simulink library "SimscapeCustomComponents_lib"  (R2025b)
settings: Solver=VariableStepAuto  StartTime=0.0  StopTime=10.0  RelTol=1e-3
undefined symbols (not defined in the file or in its folder): base, baseVdc, capacity, DiscIntNeverNeededParam, ee_sli_rtmsupport, filterInductance, freqeuncy, frequency, gcbh, gflInverter, gfmInverter, iMaxPU, Inertia, initialSOC, plantRating, solar, Ts, ups, Vac, windSystem, windTurbine
libraries: fl_lib x397, nesl_utility x171, eeGeneralControl x85, ee_lib x82, simulink x72, datacenter_lib x68, eeTransforms x38, slpidlib x24, buildingEnergy_lib x20, SimscapeFluids_lib x17, eeSinusoidalMeasurementV2 x8, eePwmGenerator x8
(part 17 of 24)

== system SimscapeCustomComponents_lib/Microgrid and Renewables/Control/Renewables/Power Reference Controller/PLL & Measurements/Subsystem ==
  Vabc : Inport
  Iabc : Inport  Port=2
  Demux : Demux  Outputs=3
  Demux1 : Demux  Outputs=3
  Park Transform : eeTransforms/Park Transform  AxisAlignment=Q-axis  PowerInvariant=off
  Park Transform1 : eeTransforms/Park Transform  AxisAlignment=Q-axis  PowerInvariant=off
  Scope : Scope  NumInputPorts=2
      settings: ActiveDisplayYMinimum=0.97158  ActiveDisplayYMaximum=1.00612  DataLoggingVariableName=ScopeData5
  "Sinusoidal Measurement (PLL, Three-Phase)" : eeSinusoidalMeasurementV2/Sinusoidal Measurement (PLL, Three-Phase)  InputFilter=on  InputNormalization=off  Kp_LF=kpPLL  Ki_LF=kiPLL  F0=frequency  Theta0=0  Ts=-1
  Terminator : Terminator
  Terminator1 : Terminator
  mag : Outport
  freq : Outport  Port=2
  angle : Outport  Port=3
  Vd : Outport  Port=4
  Vq : Outport  Port=5
  Id1 : Outport  Port=6
  Iq1 : Outport  Port=7
  wires:
  Demux/3 -> Terminator/1
  Vabc/1 -> Park Transform/1, "Sinusoidal Measurement (PLL, Three-Phase)"/1
  Park Transform/1 -> Demux/1
  Demux/1 -> Scope/1, Vd/1
  Demux/2 -> Scope/2, Vq/1
  "Sinusoidal Measurement (PLL, Three-Phase)"/2 -> angle/1, Park Transform1/2, Park Transform/2
  "Sinusoidal Measurement (PLL, Three-Phase)"/1 -> freq/1
  "Sinusoidal Measurement (PLL, Three-Phase)"/3 -> mag/1
  Park Transform1/1 -> Demux1/1
  Demux1/1 -> Id1/1
  Demux1/2 -> Iq1/1
  Demux1/3 -> Terminator1/1
  Iabc/1 -> Park Transform1/1

== system SimscapeCustomComponents_lib/Microgrid and Renewables/Control/Renewables/Power Reference Controller/Power Reference Controller/Current_controller ==
  id-ref : Inport
  ipvd : Inport  Port=2
  iqref : Inport  Port=3
  iq : Inport  Port=4
  Vd : Inport  Port=5
  Vq : Inport  Port=6
  Constant4 : Constant  Value=0
  Gain1 : Gain  Gain=2*1*pi*60*L/zbase
  Gain2 : Gain  Gain=2*1*pi*60*L/zbase
  Mux1 : Mux  Inputs=3
  PID Controller : slpidlib/PID Controller  Controller=PID  Form=Parallel  TimeDomain=Discrete-time  UseExternalTs=off  SampleTime=-1  IntegratorMethod=Forward Euler  FilterMethod=Forward Euler  ControllerParametersSource=internal  P=Kpic  I=Kiic  UseKiTs=off  D=Kd  UseExternalDerivativeSource=off  N=100  UseFilter=on  TunerSelectOption=Transfer Function Based (PID Tuner App)  InitialConditionSource=internal  InitialConditionForIntegrator=0  InitialConditionForFilter=0  DifferentiatorICPrevScaledInput=0  ExternalReset=none  TrackingMode=off  Kt=1  LimitOutput=on  SatLimitsSource=internal  UpperSaturationLimit=3  LowerSaturationLimit=-3  LinearizeAsGain=on  AntiWindupMode=clamping  Kb=1  LimitIntegrator=on  UpperIntegratorSaturationLimit=3  LowerIntegratorSaturationLimit=-3  POutMin=[]  POutMax=[]  IOutMin=[]  IOutMax=[]  DOutMin=[]  DOutMax=[]  NOutMin=[]  NOutMax=[]  SumOutMin=[]  SumOutMax=[]  SaturationOutMin=[]  SaturationOutMax=[]  PParamMin=[]  PParamMax=[]  IParamMin=[]  IParamMax=[]  DParamMin=[]  DParamMax=[]  NParamMin=[]  NParamMax=[]  KbParamMin=[]  KbParamMax=[]  KtParamMin=[]  KtParamMax=[]  KbOutMin=[]  KbOutMax=[]  KtOutMin=[]  KtOutMax=[]  IntegratorOutMin=[]  IntegratorOutMax=[]  FilterOutMin=[]  FilterOutMax=[]  SumI1OutMin=[]  SumI1OutMax=[]  SumI2OutMin=[]  SumI2OutMax=[]  SumI3OutMin=[]  SumI3OutMax=[]  SumI4OutMin=[]  SumI4OutMax=[]  SumDOutMin=[]  SumDOutMax=[]  DifferentiatorOutMin=[]  DifferentiatorOutMax=[]  FilterDiffOutCoefMin=[]  FilterDiffOutCoefMax=[]  ReciprocalOutMin=[]  ReciprocalOutMax=[]  SumDenOutMin=[]  SumDenOutMax=[]  SumNumOutMin=[]  SumNumOutMax=[]  DivideOutMin=[]  DivideOutMax=[]  UdiffTsProdOutMin=[]  UdiffTsProdOutMax=[]  NTsProdOutMin=[]  NTsProdOutMax=[]  UintegralTsProdOutMin=[]  UintegralTsProdOutMax=[]  UngainTsProdOutMin=[]  UngainTsProdOutMax=[]  ClampingZeroOutDataTypeStr=Inherit: Inherit via back propagation  ClampingZeroOutMin=[]  ClampingZeroOutMax=[]  FilterDenConstantOutDataTypeStr=Inherit: Inherit via back propagation  FilterDenConstantOutMin=[]  FilterDenConstantOutMax=[]  PCopyOutDataTypeStr=Inherit: Inherit via back propagation  PCopyOutMin=[]  PCopyOutMax=[]  NCopyOutDataTypeStr=Inherit: Inherit via back propagation  NCopyOutMin=[]  NCopyOutMax=[]  IntegratorContinuousStateAttributes=''  IntegratorStateMustResolveToSignalObject=off  IntegratorRTWStateStorageClass=Auto  FilterContinuousStateAttributes=''  FilterStateMustResolveToSignalObject=off  FilterRTWStateStorageClass=Auto  ParallelPVariant=InternalParameters  IdealPVariant=Disabled  IVariant=InternalParameters  DVariant=InternalParameters  IntegratorVariant=Discrete  SatVariant=Enabled  AWVariant=DiscClampingParallel  PCopyVariant=Disabled  TRVariant=Disabled  FdbkBlocksVariant=Forward  IdealPFdbkVariant=Disabled  SatFdbkVariant=Disabled  DerivativeFilterVariant=ForwardEulerFilter  NVariant=InternalParameters  NCopyVariant=Disabled  FilterICVariant=InternalICsFilter  IntegratorICVariant=InternalICs  ExternalResetVariant=Disabled  TRSumVariant=Passthrough  SumFdbkVariant=Disabled  SumVariant=Sum_PID  TsampFilterVariant=InternalTs  TsampNgainVariant=Passthrough  TsampIntegralVariant=Disabled_SignalSpec  ExternalSaturationOutDataTypeStr=Inherit: Same as second input  DerivativeSourceVariant=ErrorSignal  PreIntVariant=InternalPreInt
  PID Controller1 : slpidlib/PID Controller  Controller=PID  Form=Parallel  TimeDomain=Discrete-time  UseExternalTs=off  SampleTime=-1  IntegratorMethod=Forward Euler  FilterMethod=Forward Euler  ControllerParametersSource=internal  P=Kpic  I=Kiic  UseKiTs=off  D=Kd  UseExternalDerivativeSource=off  N=100  UseFilter=on  TunerSelectOption=Transfer Function Based (PID Tuner App)  InitialConditionSource=internal  InitialConditionForIntegrator=0  InitialConditionForFilter=0  DifferentiatorICPrevScaledInput=0  ExternalReset=none  TrackingMode=off  Kt=1  LimitOutput=on  SatLimitsSource=internal  UpperSaturationLimit=3  LowerSaturationLimit=-3  LinearizeAsGain=on  AntiWindupMode=clamping  Kb=1  LimitIntegrator=on  UpperIntegratorSaturationLimit=3  LowerIntegratorSaturationLimit=-3  POutMin=[]  POutMax=[]  IOutMin=[]  IOutMax=[]  DOutMin=[]  DOutMax=[]  NOutMin=[]  NOutMax=[]  SumOutMin=[]  SumOutMax=[]  SaturationOutMin=[]  SaturationOutMax=[]  PParamMin=[]  PParamMax=[]  IParamMin=[]  IParamMax=[]  DParamMin=[]  DParamMax=[]  NParamMin=[]  NParamMax=[]  KbParamMin=[]  KbParamMax=[]  KtParamMin=[]  KtParamMax=[]  KbOutMin=[]  KbOutMax=[]  KtOutMin=[]  KtOutMax=[]  IntegratorOutMin=[]  IntegratorOutMax=[]  FilterOutMin=[]  FilterOutMax=[]  SumI1OutMin=[]  SumI1OutMax=[]  SumI2OutMin=[]  SumI2OutMax=[]  SumI3OutMin=[]  SumI3OutMax=[]  SumI4OutMin=[]  SumI4OutMax=[]  SumDOutMin=[]  SumDOutMax=[]  DifferentiatorOutMin=[]  DifferentiatorOutMax=[]  FilterDiffOutCoefMin=[]  FilterDiffOutCoefMax=[]  ReciprocalOutMin=[]  ReciprocalOutMax=[]  SumDenOutMin=[]  SumDenOutMax=[]  SumNumOutMin=[]  SumNumOutMax=[]  DivideOutMin=[]  DivideOutMax=[]  UdiffTsProdOutMin=[]  UdiffTsProdOutMax=[]  NTsProdOutMin=[]  NTsProdOutMax=[]  UintegralTsProdOutMin=[]  UintegralTsProdOutMax=[]  UngainTsProdOutMin=[]  UngainTsProdOutMax=[]  ClampingZeroOutDataTypeStr=Inherit: Inherit via back propagation  ClampingZeroOutMin=[]  ClampingZeroOutMax=[]  FilterDenConstantOutDataTypeStr=Inherit: Inherit via back propagation  FilterDenConstantOutMin=[]  FilterDenConstantOutMax=[]  PCopyOutDataTypeStr=Inherit: Inherit via back propagation  PCopyOutMin=[]  PCopyOutMax=[]  NCopyOutDataTypeStr=Inherit: Inherit via back propagation  NCopyOutMin=[]  NCopyOutMax=[]  IntegratorContinuousStateAttributes=''  IntegratorStateMustResolveToSignalObject=off  IntegratorRTWStateStorageClass=Auto  FilterContinuousStateAttributes=''  FilterStateMustResolveToSignalObject=off  FilterRTWStateStorageClass=Auto  ParallelPVariant=InternalParameters  IdealPVariant=Disabled  IVariant=InternalParameters  DVariant=InternalParameters  IntegratorVariant=Discrete  SatVariant=Enabled  AWVariant=DiscClampingParallel  PCopyVariant=Disabled  TRVariant=Disabled  FdbkBlocksVariant=Forward  IdealPFdbkVariant=Disabled  SatFdbkVariant=Disabled  DerivativeFilterVariant=ForwardEulerFilter  NVariant=InternalParameters  NCopyVariant=Disabled  FilterICVariant=InternalICsFilter  IntegratorICVariant=InternalICs  ExternalResetVariant=Disabled  TRSumVariant=Passthrough  SumFdbkVariant=Disabled  SumVariant=Sum_PID  TsampFilterVariant=InternalTs  TsampNgainVariant=Passthrough  TsampIntegralVariant=Disabled_SignalSpec  ExternalSaturationOutDataTypeStr=Inherit: Same as second input  DerivativeSourceVariant=ErrorSignal  PreIntVariant=InternalPreInt
  Saturation : Saturate  UpperLimit=1.2  LowerLimit=-1.2
  Saturation1 : Saturate  UpperLimit=1.2  LowerLimit=-1.2
  Scope : Scope  NumInputPorts=2
      settings: ActiveDisplayYMinimum=0.49995  ActiveDisplayYMaximum=0.50039
  Scope1 : Scope  NumInputPorts=2
      settings: ActiveDisplayYMinimum=-1  ActiveDisplayYMaximum=1  DataLoggingVariableName=ScopeData2
  Scope2 : Scope  NumInputPorts=3
      settings: ActiveDisplayYMinimum=0.92426  ActiveDisplayYMaximum=1.0261  DataLoggingVariableName=ScopeData2
  Sum1 : Sum  Inputs=|+-
  Sum3 : Sum  Inputs=|++-
  Sum4 : Sum  Inputs=|+++
  Sum5 : Sum  Inputs=|+-
  mdq0 : Outport
  wires:
  PID Controller/1 -> Scope2/2, Sum3/2
  Sum3/1 -> Saturation/1, [Ed]
  Gain2/1 -> Scope2/3, Sum3/3
  ipvd/1 -> Scope/2, Gain1/1, Sum1/2
  id-ref/1 -> Scope/1, Sum1/1
  Gain1/1 -> Sum4/3
  Vq/1 -> Sum4/2
  iq/1 -> Scope1/2, Gain2/1, Sum5/2
  Sum1/1 -> PID Controller/1
  Constant4/1 -> Mux1/3
  Sum5/1 -> PID Controller1/1
  PID Controller1/1 -> Sum4/1
  Sum4/1 -> Saturation1/1, [Eq]
  Mux1/1 -> mdq0/1
  iqref/1 -> Scope1/1, Sum5/1
  Saturation/1 -> Mux1/1
  Saturation1/1 -> Mux1/2
  Vd/1 -> Scope2/1, Sum3/1

== system SimscapeCustomComponents_lib/Microgrid and Renewables/Control/Renewables/Power Reference Controller/Power Reference Controller/Reference Current ==
  note: Current Limiters
  note: Avoid division by zero during start
  V-mag : Inport
  LVRT_iq : Inport  Port=2
  PRef : Inport  Port=3
  QRef : Inport  Port=4
  Constant1 : Constant
  Constant3 : Constant  Value=Imax
  Current limits : Subsystem
  Refernce id generation : Subsystem
  Refernce iq generation : Subsystem
  Switch : Switch  Criteria=u2 ~= 0  SaturateOnIntegerOverflow=off  InputSameDT=off
  Unit Delay1 : UnitDelay  SampleTime=Ts
  Unit Delay3 : UnitDelay  SampleTime=Ts
  id_ref : Outport
  iq_ref : Outport  Port=2
  wires:
  Unit Delay1/1 -> Current limits/2(iqref)
  Current limits/1(iubq) -> Refernce iq generation/1(ubiq)
  Unit Delay3/1 -> Current limits/3(idref)
  Constant3/1 -> Current limits/1(Imax)
  Refernce id generation/1(id_ref) -> id_ref/1, Unit Delay3/1
  Refernce iq generation/1(iq_ref) -> Unit Delay1/1, iq_ref/1
  LVRT_iq/1 -> Refernce iq generation/3(LVRT_iq)
  V-mag/1 -> Switch/1, Switch/2
  Switch/1 -> Refernce id generation/1(V_mag), Refernce iq generation/2(V_mag)
  Constant1/1 -> Switch/3
  QRef/1 -> Refernce iq generation/4(Q_ref)
  PRef/1 -> Refernce id generation/3(PRef)
  Current limits/2(iubd) -> Refernce id generation/2(ubid)

== system SimscapeCustomComponents_lib/Microgrid and Renewables/Control/Renewables/Solar PV Controller/DC voltage controller & current reference/Current limits ==
  Imax : Inport
  idref : Inport  Port=2
  Sqrt1 : Sqrt
  Square3 : Math  Operator=square
  Square4 : Math  Operator=square
  Sum9 : Sum  Inputs=|+-
  iubd : Outport
  iubq : Outport  Port=2
  wires:
  Sum9/1 -> Sqrt1/1
  Square3/1 -> Sum9/1
  Square4/1 -> Sum9/2
  Imax/1 -> iubd/1, Square3/1
  Sqrt1/1 -> iubq/1
  idref/1 -> Square4/1

== system SimscapeCustomComponents_lib/Microgrid and Renewables/Control/Renewables/Solar PV Controller/DC voltage controller & current reference/If Action Subsystem ==
  note: iq_ref_generator
  note: id_ref_generator
  Q ref : Inport
  Vmag : Inport  Port=2
  P pv : Inport  Port=3
  vdc : Inport  Port=4
  vdc ref : Inport  Port=5
  Action Port : ActionPort
  Subsystem : Subsystem
  Subsystem1 : Subsystem
  iq ref : Outport
  id ref : Outport  Port=2
  wires:
  [ubid] -> Subsystem1/5(id ub)
  [ubiq] -> Subsystem/2(iq ub)
  P pv/1 -> Subsystem1/2(P pv)
  Q ref/1 -> Subsystem/3(Q ref)
  vdc/1 -> Subsystem1/3(vdc)
  Vmag/1 -> Subsystem1/1(Vmag), Subsystem/1(V mag)
  vdc ref/1 -> Subsystem1/4(vdc ref)
  Subsystem1/1(idref) -> id ref/1
  Subsystem/1(iqref) -> iq ref/1

== system SimscapeCustomComponents_lib/Microgrid and Renewables/Control/Renewables/Solar PV Controller/DC voltage controller & current reference/Subsystem ==
  V mag : Inport
  iq ub : Inport  Port=2
  Q ref : Inport  Port=3
  Constant : Constant  Value=1e-3
  Data Type Conversion Inherited : simulink/Signal Attributes/Data Type Conversion Inherited  ConvertRealWorld=Real World Value  DoSatur=off
  Divide2 : Product  Inputs=*/
  Gain1 : Gain  Gain=-1
  Gain3 : Gain  Gain=-1
  Saturation Dynamic2 : simulink/Discontinuities/Saturation Dynamic  OutMin=[]  OutMax=[]  OutDataTypeStr=Inherit: Same as second input  OutDataType=fixdt(1, 16)  OutScaling=2^-10  DoSatur=off
  Scope : Scope  NumInputPorts=3
      settings: ActiveDisplayYMinimum=1.32868  ActiveDisplayYMaximum=1.39248  DataLoggingVariableName=ScopeData8
  Switch : Switch  Criteria=u2 ~= 0  SaturateOnIntegerOverflow=off  InputSameDT=off
  iq ub1 : InportShadow  Port=2
  iqref : Outport
  wires:
  iq ub1/1 -> Gain3/1
  Divide2/1 -> Saturation Dynamic2/2, Scope/2
  Q ref/1 -> Divide2/1
  Gain3/1 -> Saturation Dynamic2/3, Scope/3
  iq ub/1 -> Saturation Dynamic2/1, Scope/1
  Saturation Dynamic2/1 -> Gain1/1
  V mag/1 -> Data Type Conversion Inherited/1, Switch/2, Switch/1
  Switch/1 -> Divide2/2
  Constant/1 -> Data Type Conversion Inherited/2
  Data Type Conversion Inherited/1 -> Switch/3
  Gain1/1 -> iqref/1

== system SimscapeCustomComponents_lib/Microgrid and Renewables/Control/Renewables/Solar PV Controller/DC voltage controller & current reference/Subsystem1 ==
  Vmag : Inport
  P pv : Inport  Port=2
  vdc : Inport  Port=3
  vdc ref : Inport  Port=4
  id ub : Inport  Port=5
  Constant : Constant  Value=1e-3
  Constant4 : Constant  Value=0
  Data Type Conversion Inherited : simulink/Signal Attributes/Data Type Conversion Inherited  ConvertRealWorld=Real World Value  DoSatur=off
  Divide : Product  Inputs=/*
  Gain4 : Gain  Gain=1/(mVAbase)
  Saturation Dynamic1 : simulink/Discontinuities/Saturation Dynamic  OutMin=[]  OutMax=[]  OutDataTypeStr=Inherit: Same as second input  OutDataType=fixdt(1, 16)  OutScaling=2^-10  DoSatur=off
  Scope : Scope  NumInputPorts=2
      settings: ActiveDisplayYMinimum=715.83213  ActiveDisplayYMaximum=1444.49375
  Scope1 : Scope  NumInputPorts=3
      settings: ActiveDisplayYMinimum=0.2  ActiveDisplayYMaximum=2.2  DataLoggingVariableName=ScopeData7
  Sum : Sum  Inputs=|++
  Switch : Switch  Criteria=u2 ~= 0  SaturateOnIntegerOverflow=off  InputSameDT=off
  V_dc_Controller1 : Subsystem
  idref : Outport
  wires:
  Constant4/1 -> Saturation Dynamic1/3
  P pv/1 -> Gain4/1
  V_dc_Controller1/1(Out1) -> Sum/2
  Sum/1 -> Saturation Dynamic1/2, Scope1/2
  vdc ref/1 -> V_dc_Controller1/2(vdc ref), Scope/2
  id ub/1 -> Scope1/1, Saturation Dynamic1/1
  Gain4/1 -> Divide/2
  Divide/1 -> Sum/1
  Saturation Dynamic1/1 -> idref/1, Scope1/3
  vdc/1 -> V_dc_Controller1/1(vdc), Scope/1
  Vmag/1 -> Data Type Conversion Inherited/1, Switch/2, Switch/1
  Switch/1 -> Divide/1
  Constant/1 -> Data Type Conversion Inherited/2
  Data Type Conversion Inherited/1 -> Switch/3

== system SimscapeCustomComponents_lib/Microgrid and Renewables/Control/Renewables/Solar PV Controller/PLL & Measurements/Subsystem ==
  abc : Inport
  Demux : Demux  Outputs=3
  Park Transform : eeTransforms/Park Transform  AxisAlignment=Q-axis  PowerInvariant=off
  "Sinusoidal Measurement (PLL, Three-Phase)" : eeSinusoidalMeasurementV2/Sinusoidal Measurement (PLL, Three-Phase)  InputFilter=on  InputNormalization=off  Kp_LF=Kppll  Ki_LF=Kipll  F0=frequency  Theta0=initialPhase  Ts=sampleTime
  Terminator : Terminator
  mag : Outport
  freq : Outport  Port=2
  angle : Outport  Port=3
  Vd : Outport  Port=4
  Vq : Outport  Port=5
  wires:
  "Sinusoidal Measurement (PLL, Three-Phase)"/2 -> angle/1, Park Transform/2
  Demux/3 -> Terminator/1
  abc/1 -> Park Transform/1, "Sinusoidal Measurement (PLL, Three-Phase)"/1
  Park Transform/1 -> Demux/1
  Demux/1 -> Vd/1
  Demux/2 -> Vq/1
  "Sinusoidal Measurement (PLL, Three-Phase)"/1 -> freq/1
  "Sinusoidal Measurement (PLL, Three-Phase)"/3 -> mag/1

== system SimscapeCustomComponents_lib/Microgrid and Renewables/Control/Renewables/Solar PV Controller/Variant Subsystem/INC MPP ==
  Ipv : Inport
  Vpv : Inport  Port=2
  Abs : Abs  SaturateOnIntegerOverflow=off
  Add : Sum
  Constant : Constant  Value=0  SampleTime=sampleTime
  Constant1 : Constant  Value=delV  SampleTime=sampleTime
  Data Type Conversion Inherited : simulink/Signal Attributes/Data Type Conversion Inherited  ConvertRealWorld=Real World Value  DoSatur=off
  Data Type Conversion Inherited1 : simulink/Signal Attributes/Data Type Conversion Inherited  ConvertRealWorld=Real World Value  DoSatur=off
  Divide : Product  Inputs=*/
  Divide1 : Product  Inputs=*/
  Filtered Derivative (Discrete or Continuous) : eeGeneralControl/Filtered Derivative (Discrete or Continuous)  K=1  T=tSettling*2  B=inf  A=-inf  minRatio=1  init_option=Inherited from block input  x0=0  Ts=sampleTime
  Filtered Derivative (Discrete or Continuous)1 : eeGeneralControl/Filtered Derivative (Discrete or Continuous)  K=1  T=tSettling*2  B=inf  A=-inf  minRatio=1  init_option=Inherited from block input  x0=0  Ts=sampleTime
  Subtract5 : Sum  Inputs=-+
  Sum2 : Sum  Inputs=|++
  Switch : Switch  Criteria=u2 ~= 0  SaturateOnIntegerOverflow=off  InputSameDT=off
  Switch1 : Switch  Criteria=u2 > Threshold  SaturateOnIntegerOverflow=off  InputSameDT=off
  Switch4 : Switch  Criteria=u2 > Threshold  Threshold=1e-2  SaturateOnIntegerOverflow=off  InputSameDT=off
  Switch5 : Switch  Criteria=u2 > Threshold  SaturateOnIntegerOverflow=off  InputSameDT=off
  start MPPT Voltage : Constant  Value=Vdc  SampleTime=sampleTime
  Vmpp : Outport  VectorParamsAs1DForOutWhenUnconnected=off
  wires:
  Ipv/1 -> Filtered Derivative (Discrete or Continuous)/1, Divide1/1
  Switch5/1 -> Data Type Conversion Inherited1/1, Add/1, Subtract5/2
  Vpv/1 -> Filtered Derivative (Discrete or Continuous)1/1, Divide1/2, Data Type Conversion Inherited/1, Switch5/2, Switch5/1
  Add/1 -> [Vinc]  "INC"
  Subtract5/1 -> [Vdec]  "DEC"
  Filtered Derivative (Discrete or Continuous)/1 -> Switch/3, Divide/1
  Divide/1 -> Sum2/1
  Divide1/1 -> Sum2/2
  Sum2/1 -> Switch/1
  Switch/1 -> Switch1/2, Abs/1
  [Vinc] -> Switch1/1
  [Vdec] -> Switch1/3
  Filtered Derivative (Discrete or Continuous)1/1 -> Switch/2, Divide/2
  Abs/1 -> Switch4/2
  Constant/1 -> Switch4/3
  Constant1/1 -> Switch4/1
  Switch1/1 -> Vmpp/1
  Data Type Conversion Inherited/1 -> Switch5/3
  start MPPT Voltage/1 -> Data Type Conversion Inherited/2
  Switch4/1 -> Data Type Conversion Inherited1/2
  Data Type Conversion Inherited1/1 -> Add/2, Subtract5/1

== system SimscapeCustomComponents_lib/Microgrid and Renewables/Control/Renewables/Solar PV Controller/Variant Subsystem/P&O MPP ==
  Ipv : Inport
  Vpv : Inport  Port=2
  AND1 : Logic  IconShape=distinctive  AllPortsSameDT=off  OutDataTypeStr=boolean
  Add : Sum
  Compare To Zero1 : simulink/Logic and Bit Operations/Compare To Zero  relop=>=  OutDataTypeStr=boolean
  Compare To Zero2 : simulink/Logic and Bit Operations/Compare To Zero  relop=>=  OutDataTypeStr=boolean
  Constant1 : Constant  Value=delV  SampleTime=sampleTime
  Data Type Conversion Inherited : simulink/Signal Attributes/Data Type Conversion Inherited  ConvertRealWorld=Real World Value  DoSatur=off
  Data Type Conversion Inherited1 : simulink/Signal Attributes/Data Type Conversion Inherited  ConvertRealWorld=Real World Value  DoSatur=off
  Filtered Derivative (Discrete or Continuous) : eeGeneralControl/Filtered Derivative (Discrete or Continuous)  K=1  T=tSettling*2  B=inf  A=-inf  minRatio=1  init_option=Inherited from block input  x0=0  Ts=sampleTime
  Filtered Derivative (Discrete or Continuous)1 : eeGeneralControl/Filtered Derivative (Discrete or Continuous)  K=1  T=tSettling*2  B=inf  A=-inf  minRatio=1  init_option=Inherited from block input  x0=0  Ts=sampleTime
  NOR : Logic  Operator=NOR  IconShape=distinctive  AllPortsSameDT=off  OutDataTypeStr=boolean
  OR : Logic  Operator=OR  IconShape=distinctive  AllPortsSameDT=off  OutDataTypeStr=boolean
  Product : Product
  Subtract5 : Sum  Inputs=-+
  Switch4 : Switch  Criteria=u2 ~= 0  SaturateOnIntegerOverflow=off  InputSameDT=off
  Switch5 : Switch  Criteria=u2 > Threshold  SaturateOnIntegerOverflow=off  InputSameDT=off
  start MPPT Voltage : Constant  Value=Vdc  SampleTime=sampleTime
  Vmpp : Outport  VectorParamsAs1DForOutWhenUnconnected=off
  wires:
  OR/1 -> Switch4/2
  Compare To Zero1/1 -> NOR/1, AND1/2
  Compare To Zero2/1 -> NOR/2, AND1/1
  Switch5/1 -> Data Type Conversion Inherited1/1, Add/1, Subtract5/2
  Constant1/1 -> Data Type Conversion Inherited1/2
  Vpv/1 -> Product/2, Filtered Derivative (Discrete or Continuous)1/1, Data Type Conversion Inherited/1, Switch5/2, Switch5/1
  Add/1 -> [Vinc]  "INC"
  NOR/1 -> OR/2
  Subtract5/1 -> [Vdec]  "DEC"
  [Vdec] -> Switch4/3
  Filtered Derivative (Discrete or Continuous)1/1 -> Compare To Zero1/1
  Filtered Derivative (Discrete or Continuous)/1 -> Compare To Zero2/1
  AND1/1 -> OR/1
  [Vinc] -> Switch4/1
  Ipv/1 -> Product/1
  Product/1 -> Filtered Derivative (Discrete or Continuous)/1
  Switch4/1 -> Vmpp/1
  Data Type Conversion Inherited/1 -> Switch5/3
  start MPPT Voltage/1 -> Data Type Conversion Inherited/2
  Data Type Conversion Inherited1/1 -> Add/2, Subtract5/1

== system SimscapeCustomComponents_lib/Microgrid and Renewables/Control/Renewables/Wind Controller/Machine Converter Control/Measurements ==
  iabc_sens : Inport
  w_sens : Inport  Port=2
  th_sens : Inport  Port=3
  Vdc_sens : Inport  Port=4
  2*pi : Constant  Value=2*pi  SampleTime=-1
  Math Function : Math  Operator=mod  SignedPower=on
  pole pairs : Gain  Gain=p
  "pole pairs " : Gain  Gain=p
  we : Outport  VectorParamsAs1DForOutWhenUnconnected=off
  iabc : Outport  Port=2  VectorParamsAs1DForOutWhenUnconnected=off
  theta : Outport  Port=3  VectorParamsAs1DForOutWhenUnconnected=off
  Vdc : Outport  Port=4  VectorParamsAs1DForOutWhenUnconnected=off
  wires:
  w_sens/1 -> pole pairs/1
  iabc_sens/1 -> iabc/1
  pole pairs/1 -> we/1
  2*pi/1 -> Math Function/2
  th_sens/1 -> "pole pairs "/1
  "pole pairs "/1 -> Math Function/1
  Vdc_sens/1 -> Vdc/1
  Math Function/1 -> theta/1

== system SimscapeCustomComponents_lib/Microgrid and Renewables/Control/Renewables/Wind Controller/Machine Converter Control/Power Controller ==
  windSpeed : Inport
  Derating Control : Subsystem
  Greater than : simulink/Logic and Bit Operations/Compare To Constant  relop=>  const=12  OutDataTypeStr=boolean
  Less than or equal to : simulink/Logic and Bit Operations/Compare To Constant  relop=<=  const=12  OutDataTypeStr=boolean
  Limiter Function Power Demand : Subsystem
  MPPT Control : Subsystem
  activePowerDemand : Outport
  wires:
  windSpeed/1 -> Greater than/1, Less than or equal to/1, MPPT Control/1(windSpeed)
  Less than or equal to/1 -> MPPT Control/Enable
  Greater than/1 -> Derating Control/Enable
  MPPT Control/1(activePowerDemand) -> Limiter Function Power Demand/1(activePowerDemandMPPT)
  Derating Control/1(activePowerDemand) -> Limiter Function Power Demand/2(activePowerDemandDerating)
  Limiter Function Power Demand/1(activePowerDemand) -> activePowerDemand/1

== system SimscapeCustomComponents_lib/Microgrid and Renewables/Control/Renewables/Wind Controller/Machine Converter Control/Subsystem ==
  note: LVRT Crowbar Control
  Vdc : Inport
  LVRT : Inport  Port=2
  Abs : Abs  SaturateOnIntegerOverflow=off
  Constant1 : Constant  Value=Vdc
  Product : Product
  Relay : Relay  OnSwitchValue=0.01001*Vdc  OffSwitchValue=0.01*Vdc
  Sum : Sum  Inputs=|+-
  Unit Delay1 : UnitDelay  SampleTime=-1
  Out1 : Outport
  wires:
  Constant1/1 -> Sum/1
  Vdc/1 -> Unit Delay1/1
  Sum/1 -> Product/1
  Abs/1 -> Relay/1
  Unit Delay1/1 -> Sum/2
  LVRT/1 -> Product/2
  Product/1 -> Abs/1
  Relay/1 -> Out1/1

== system SimscapeCustomComponents_lib/Microgrid and Renewables/Control/Renewables/Wind Controller/Wind Grid-side Converter Controller/Current_controller ==
  iWindd : Inport
  iq : Inport  Port=2
  id-ref : Inport  Port=3
  iqref : Inport  Port=4
  Vd : Inport  Port=5
  Vq : Inport  Port=6
  Constant4 : Constant  Value=0
  Gain1 : Gain  Gain=2*1*pi*frequency*inductance/baseImpedance
  Gain2 : Gain  Gain=2*1*pi*frequency*inductance/baseImpedance
  Mux1 : Mux  Inputs=3
  PI : Subsystem
  PI1 : Subsystem
  Sum1 : Sum  Inputs=|+-
  Sum3 : Sum  Inputs=|++-
  Sum4 : Sum  Inputs=|+++
  Sum5 : Sum  Inputs=|+-
  Refrence_mdq0 : Outport
  wires:
  PI/1(Out2) -> Sum3/2
  Sum3/1 -> Mux1/1, [Ed]
  Gain2/1 -> Sum3/3
  iWindd/1 -> Gain1/1, Sum1/2
  id-ref/1 -> Sum1/1
  Gain1/1 -> Sum4/3
  Vq/1 -> Sum4/2
  iq/1 -> Gain2/1, Sum5/2
  Sum1/1 -> PI/1(Input)
  Vd/1 -> Sum3/1
  Constant4/1 -> Mux1/3
  Sum5/1 -> PI1/1(Input)
  iqref/1 -> Sum5/1
  PI1/1(Out2) -> Sum4/1
  Sum4/1 -> Mux1/2, [Eq]
  Mux1/1 -> Refrence_mdq0/1  "m_dqo"

== system SimscapeCustomComponents_lib/Microgrid and Renewables/Control/Renewables/Wind Controller/Wind Grid-side Converter Controller/DC Bus Chopper control  ==
  note: LVRT Detection
  In1 : Inport
  Constant1 : Constant
  Constant2 : Constant  Value=0
  Switch : Switch  Criteria=u2 > Threshold  Threshold=0.9  SaturateOnIntegerOverflow=off  InputSameDT=off
  Unit Delay : UnitDelay  SampleTime=-1
  Out1 : Outport
  wires:
  Switch/1 -> Out1/1
  Constant1/1 -> Switch/3
  Constant2/1 -> Switch/1
  In1/1 -> Unit Delay/1
  Unit Delay/1 -> Switch/2

== system SimscapeCustomComponents_lib/Microgrid and Renewables/Control/Renewables/Wind Controller/Wind Grid-side Converter Controller/DC voltage controller & current reference ==
  note: Limiter
  note: iq_ref_generator
  note: id_ref_generator
  Q_ref : Inport
  Vmag : Inport  Port=2
  Wind_Mpp_vdc : Inport  Port=3
  Wind_vdc : Inport  Port=4
  lvrt.iq : Inport  Port=5
  Constant : Constant
  Constant1 : Constant  Value=iMaxPU
  Current limits : Subsystem
  Subsystem : Subsystem
  Subsystem1 : Subsystem
  Switch : Switch  Criteria=u2 > Threshold  SaturateOnIntegerOverflow=off  InputSameDT=off
  Unit Delay1 : UnitDelay  SampleTime=Ts
  Unit Delay3 : UnitDelay  SampleTime=Ts
  id_ref : Outport
  iq_ref : Outport  Port=2
  wires:
  Current limits/2(iubd) -> Subsystem1/3(id_ub)
  Subsystem/1(Out1) -> Unit Delay1/1, iq_ref/1
  Constant1/1 -> Current limits/1(Imax)
  Unit Delay1/1 -> Current limits/2(iqref)
  Subsystem1/1(Out1) -> id_ref/1, Unit Delay3/1
  Unit Delay3/1 -> Current limits/3(idref)
  Q_ref/1 -> Subsystem/4(Q_ref)
  Wind_Mpp_vdc/1 -> Subsystem1/1(Wind_Mpp_vdc)
  Wind_vdc/1 -> Subsystem1/2(Wind_vdc)
  Current limits/1(iubq) -> Subsystem/2(iq_ub)
  lvrt.iq/1 -> Subsystem/3(lvrt.iq)
  Vmag/1 -> Switch/1, Switch/2
  Switch/1 -> Subsystem/1(V_mag)
  Constant/1 -> Switch/3

== system SimscapeCustomComponents_lib/Microgrid and Renewables/Sources/Generator Integrated/Detailed/Governor and Prime Mover /Governor ==
  pu_velocity : Inport
  PRef : Inport  Port=2
  1/T_G : Gain  Gain=1/T_G
  1/droop : Gain  Gain=1/(droop_percentage/100)
  Delta load setpoint : Sum  Inputs=+-|
  Delta speed : Sum  Inputs=-+|
  Discrete-Time Integrator1 : DiscreteIntegrator  InitialCondition=pu_torque0  SampleTime=-1  ICPrevOutput=DiscIntNeverNeededParam  ICPrevScaledInput=DiscIntNeverNeededParam
  Scope : Scope  NumInputPorts=2
  Scope1 : Scope  NumInputPorts=2
  Speed_ref : Constant  Value=pu_speed_reference
  Subtract : Sum  Inputs=|+-
  delta_y : Outport  VectorParamsAs1DForOutWhenUnconnected=off
  wires:
  Speed_ref/1 -> Delta speed/1
  Delta speed/1 -> Scope/1, 1/droop/1
  pu_velocity/1 -> Scope/2, Delta speed/2
  1/droop/1 -> Delta load setpoint/2
  Delta load setpoint/1 -> Subtract/1
  Subtract/1 -> Scope1/1, 1/T_G/1
  1/T_G/1 -> Discrete-Time Integrator1/1
  Discrete-Time Integrator1/1 -> Scope1/2, delta_y/1, Subtract/2
  PRef/1 -> Delta load setpoint/1

== system SimscapeCustomComponents_lib/Microgrid and Renewables/Sources/Generator Integrated/Detailed/Governor and Prime Mover /Non-reheat turbine ==
  delta_y : Inport
  1/T_CH : Gain  Gain=1/T_CH
  Discrete-Time Integrator1 : DiscreteIntegrator  InitialCondition=pu_torque0  SampleTime=-1  ICPrevOutput=DiscIntNeverNeededParam  ICPrevScaledInput=DiscIntNeverNeededParam
  Scope : Scope  NumInputPorts=2
  Sum : Sum  Inputs=|+-
  torque : Outport  VectorParamsAs1DForOutWhenUnconnected=off
  wires:
  delta_y/1 -> Scope/2, Sum/1
  Sum/1 -> 1/T_CH/1
  1/T_CH/1 -> Discrete-Time Integrator1/1
  Discrete-Time Integrator1/1 -> Sum/2, Scope/1, torque/1

== system SimscapeCustomComponents_lib/Microgrid and Renewables/Sources/Solar Plant/Converter/Switching/Pulse Generation ==
  G : Inport
  Constant : Constant  Value=5
  Subtract : Sum  Inputs=-+
  G1 : Outport  VectorParamsAs1DForOutWhenUnconnected=off
  G2 : Outport  Port=2  VectorParamsAs1DForOutWhenUnconnected=off
  wires:
  Subtract/1 -> G2/1
  Constant/1 -> Subtract/2
  G/1 -> G1/1, Subtract/1

== system SimscapeCustomComponents_lib/Microgrid and Renewables/Sources/Solar Plant Integrated/Detailed/PV Plant & Controller/Controller ==
  Qref : Inport
  ipv (A) : Inport  Port=2
  vdc (V) : Inport  Port=3
  Vabc : Inport  Port=4
  Iabc : Inport  Port=5
  Pref : Inport  Port=6
  Mode : Inport  Port=7
  If : If
  MPPT : Subsystem  TreatAsAtomicUnit=on
  Merge : Merge
  Power Reference : Subsystem  TreatAsAtomicUnit=on
  vabcRef (pu) : Outport
  wires:
  Mode/1 -> If/1
  Merge/1 -> vabcRef (pu)/1
  Power Reference/1(mabc) -> Merge/2
  MPPT/1(mabc) -> Merge/1
  If/2 -> Power Reference/Action
  If/1 -> MPPT/Action
  Vabc/1 -> MPPT/4(Vabc), Power Reference/2(Vabc)
  Pref/1 -> Power Reference/3(PRef)
  Iabc/1 -> MPPT/5(Iabc), Power Reference/1(Iabc)
  Qref/1 -> Power Reference/4(QRef), MPPT/1(Qref)
  vdc (V)/1 -> MPPT/3(vdc (V))
  ipv (A)/1 -> MPPT/2(ipv (A))

== system SimscapeCustomComponents_lib/Microgrid and Renewables/Sources/Solar Plant Integrated/Detailed/PV Plant & Controller/PV Plant ==
  mabc : Inport
  Converter : Subsystem  InitFcn=%solar.mask.restoreConverterLink(gcb);  Variant=on  VariantControlMode=label  LabelModeActiveChoice=Switching  mask{converterFidelity=Switching, fSw=fSw}
      mask prompts: converterFidelity "Converter Fidelity"; fSw "Switching Frequency (kHz)"
      settings: PreSaveFcn=%solar.mask.restoreConverterLink  CloseFcn=%solar.mask.restoreConverterLink
      mask TypeOptions converterFidelity: Average | Switching
      mask Callback converterFidelity: component.mask.converterFidelity(gcb);
      mask DialogControl editSwitch Prompt: Edit converter parameters
      mask DialogControl editSwitch Callback:
      | converterFidelity = get_param(gcb,'converterFidelity');
      | blockPath = [gcb,'/',converterFidelity,'/','Converter'];
      | component.mask.openBlock(blockPath);
  Current Sensor : fl_lib/Electrical/Electrical Sensors/Current Sensor
  DC- Capacitor : fl_lib/Electrical/Electrical Elements/Capacitor  c=capDC F  r=1e-6 Ohm  g=0 1/Ohm  i_specify=off  i_priority=None  i=0 A  i_nominal_specify=off  i_nominal_value=1  i_nominal_unit=A  v_specify=off  v_priority=None  v=6560*.5 V  v_nominal_specify=off  v_nominal_value=1  v_nominal_unit=V  vc_specify=on  vc_priority=None  vc=ceil(Vac*sqrt(2)*1.2) V  vc_nominal_specify=off  vc_nominal_value=1  vc_nominal_unit=V
  ERef1 : fl_lib/Electrical/Electrical Elements/Electrical Reference
  PS-Simulink Converter : nesl_utility/PS-Simulink Converter  PhysicalDomain=network_engine_domain  SubClassName=ps_output  LeftPortType=input  RightPortType=output  PseudoPeriodic=off  Frequencies=[]  VectorFormat=inherit  Unit=inherit  AffineConversion=off
  PS-Simulink Converter1 : nesl_utility/PS-Simulink Converter  PhysicalDomain=network_engine_domain  SubClassName=ps_output  LeftPortType=input  RightPortType=output  PseudoPeriodic=off  Frequencies=[]  VectorFormat=inherit  Unit=inherit  AffineConversion=off
  PV Array : ee_lib/Sources/Solar Cell  PartSpecification="{\"CollectionId\":\"SimscapeElectrical\",\"DatasetId\":\"Tata_Power_Solar|TP300|simscape.electrical.solarCell\",\"DisplayName\":\"Tata_Power_Solar:TP300\"}"  prm=ee.enum.sources.solar_cell_prm.fiveParameter  Isc=8.71 % Datasheet derived A  Voc=0.62223 % Datasheet derived V  Is=1.08146075786774e-06 % Datasheet derived A  Is2=5.42602984007438e-09 % Datasheet derived A  Iph=8.71000410148422 % Datasheet derived A  Ir0=1000 % Datasheet derived W/m^2  ec=1.52301308864556 % Datasheet derived  N2=1.87068753668451 % Datasheet derived  Rs=0.000339119125335165 % Datasheet derived Ohm  Rp=655.536158839936 % Datasheet derived Ohm  N_series=72*nSeries% Datasheet derived  N_parallel=1*nParallel % Datasheet derived  TIPH1=0.000579985599628516 % Datasheet derived 1/K  EG=1.12 % Datasheet derived eV  TXIS1=3.78147935095899 % Datasheet derived  TXIS2=12.1162776751811 % Datasheet derived  TRS1=0.141899818875295 % Datasheet derived  TRP1=0 % Parameter not set  Tmeas=25 % Datasheet derived degC  TFIXED=25 % Datasheet derived degC  thermal_mass=100 % Parameter not set J/K  initial_temperature=25 degC
      settings: AttributesFormatString=Tata_Power_Solar:TP300
  Voltage Sensor : fl_lib/Electrical/Electrical Sensors/Voltage Sensor
  ABC : PMIOPort  Side=Right
  Ir : PMIOPort  Port=2  Side=Left
  I : Outport
  V : Outport  Port=2
  wires:
  mabc/1 -> Converter/1(mabc)
  PS-Simulink Converter1/1 -> V/1
  PS-Simulink Converter/1 -> I/1
  connections:
  Voltage Sensor/RConn2 -- PV Array/RConn1 -- ERef1/LConn1 -- Converter/LConn2 -- DC- Capacitor/RConn1
  Voltage Sensor/LConn1 -- Current Sensor/RConn2 -- Converter/LConn1 -- DC- Capacitor/LConn1
  PS-Simulink Converter1/LConn1 -- Voltage Sensor/RConn1
  PS-Simulink Converter/LConn1 -- Current Sensor/RConn1
  Ir/RConn1 -- PV Array/LConn1
  ABC/RConn1 -- Converter/RConn1
  PV Array/LConn2 -- Current Sensor/LConn1

== system SimscapeCustomComponents_lib/Microgrid and Renewables/Sources/Solar Plant Integrated/Detailed/PV Plant & Controller/Sensor Dynamics ==
  Iin : Inport
  Vin : Inport  Port=2
  Current Measurement : Subsystem
  Product : Product
  Scope : Scope
      settings: ActiveDisplayYMinimum=-1.17977100562E+6  ActiveDisplayYMaximum=5.50264896669E+6  DataLoggingVariableName=ScopeData5
  Voltage Measurement : Subsystem
  I : Outport
  V : Outport  Port=2
  wires:
  Product/1 -> Scope/1
  Voltage Measurement/1(I) -> V/1, Product/1
  Vin/1 -> Voltage Measurement/1(u)
  Iin/1 -> Current Measurement/1(u)
  Current Measurement/1(V) -> I/1, Product/2

== system SimscapeCustomComponents_lib/Microgrid and Renewables/Sources/Wind Plant/Back-to-Back Converters/Switching/Grid Side Converter ==
  mabc : Inport
  Add : Sum
  Constant1 : Constant
  Converter : ee_lib/Semiconductors & Converters/Converters/Converter (Three-Phase)  port_option=ee.enum.threePhasePort.composite  fidelity_option=ee.enum.converters.fidelity.detailed  device_type=ee.enum.converters.switchingdevice.ideal  showThermalPort=false  K=0  Vth=1 V  Vgt=1 V  Vgt_off=-1 V  Ih=1 A  Vf=0.8 V  Ron=0.001 Ohm  Rds=0.001 Ohm  Goff=1e-6 1/Ohm  Eon_scalar=22.86e-3 J  Eoff_scalar=17.14e-3 J  Eoff_natural_commutation=10e-3 J  Voff=300 V  Iout_scalar=600 A  onCurrentMeasDelay=0 s  useCurrentFromPreviousCycle=false  useVoltageFromPreviousCycle=false  diode_param=ee.enum.converters.protectiondiode.nodynamics  diode_Vf=0.01 V  diode_Ron=0.0001 Ohm  diode_Goff=1e-5 1/Ohm  diode_C=50 nF  diode_iRM=-235 A  diode_iF=300 A  diode_idot=-50 A/us  diode_trr_param=ee.enum.converters.diodetrr.trr_factor  diode_trr_factor=3  diode_trr=15 us  diode_Qrr=1500 s*uA  diode_rec_loss_model=ee.enum.diode.reverseRecoveryModel.fixed  diode_ErecVal=0 J  diode_scaleWithIandV=false  diode_ErecMat=zeros(2, 3) J  diode_TjrecVec=[298.15, 398.15] K  diode_IfrecVec=[.1, 1, 10] A  diode_IrecVal=10 A  diode_VrecVal=10 V  diode_tFilter=1 / 1000 / 100 s  thermal_network_parameterization=ee.enum.thermalNetworkTopology.external  Rth=[.08, .5] K/W  Rth_Cauer=[.08, .1, .5] K/W  Rth_Foster=[.08, .14, .22, .16] K/W  thermal_mass_parameterization=ee.enum.thermalNetwork.timeconstant  thermal_mass=[.01, .5] J/K  thermal_mass_Cauer=[.01, .1, .5] J/K  thermal_mass_Foster=[.001, .005, .05, .5] J/K  thermal_time_constant=[.001, .2] s  thermal_time_constant_Cauer=[.001, .1, .2] s  thermal_time_constant_Foster=[7e-05, .0007, .01, .08] s  thermal_mass_initial_temperatures=[25, 25] degC  thermal_mass_initial_temperatures_Cauer=[25, 25, 25] degC  junction_thermal_mass=0.01 J/K  Tvec_initial_Foster=[25, 25, 25, 25] degC  snubber_type=ee.enum.converters.snubber.exclude  Cs=1e-7 F  Rs=0.1 Ohm  Vce_loss=[0, 150, 300] V
  Demux : Demux  Outputs=3
  Demux1 : Demux  Outputs=3
  Gain : Gain  Gain=5
  Gain1 : Gain  Gain=0.5
  PWM Generator : eePwmGenerator/PWM Generator  CarrCount=Up  Tper=1/(fSw*1000)  Tdelay=0  Ts=1/(10*fSw*1000)
  Pulse Generation1 : Subsystem
  Rate Transition1 : RateTransition  OutPortSampleTime=1/(10*fSw*1000)
  Simulink-PS Converter{1..6} (6 alike) : nesl_utility/Simulink-PS Converter  PhysicalDomain=network_engine_domain  SubClassName=ps_input  LeftPortType=input  RightPortType=output  PseudoPeriodic=off  Frequencies=[]  NoiseDistribution=none  NoiseParameters=[]  Unit=1  AffineConversion=off  FilteringAndDerivatives=provide  SimscapeFilterOrder=1  InputFilterTimeConstant=0.001  UdotUserProvided=0
  Six-Pulse Gate Multiplexer : ee_lib/Semiconductors & Converters/Converters/Six-Pulse Gate Multiplexer  port_option=ee.enum.controlport.ps
  + : PMIOPort  Side=Left
  - : PMIOPort  Port=2  Side=Left
  ~ : PMIOPort  Port=3  Side=Right
  wires:
  [BL] -> Simulink-PS Converter3/1
  Pulse Generation1/1(G1) -> Demux/1
  Pulse Generation1/2(G2) -> Demux1/1
  Demux1/1 -> [AL]
  Gain/1 -> Pulse Generation1/1(G)
  mabc/1 -> Add/1
  Demux/2 -> [BH]
  Demux1/2 -> [BL]
  Gain1/1 -> Rate Transition1/1
  PWM Generator/1 -> Gain/1
  [AL] -> Simulink-PS Converter5/1
  [CL] -> Simulink-PS Converter1/1
  Demux1/3 -> [CL]
  [BH] -> Simulink-PS Converter4/1
  Rate Transition1/1 -> PWM Generator/1
  [AH] -> Simulink-PS Converter6/1
  Demux/3 -> [CH]
  Constant1/1 -> Add/2
  Add/1 -> Gain1/1
  Demux/1 -> [AH]
  [CH] -> Simulink-PS Converter2/1
  connections:
  Simulink-PS Converter1/RConn1 -- Six-Pulse Gate Multiplexer/LConn6
  Six-Pulse Gate Multiplexer/LConn4 -- Simulink-PS Converter3/RConn1
  ~/RConn1 -- Converter/LConn2
  Six-Pulse Gate Multiplexer/RConn1 -- Converter/LConn1
  Six-Pulse Gate Multiplexer/LConn2 -- Simulink-PS Converter5/RConn1
  Six-Pulse Gate Multiplexer/LConn3 -- Simulink-PS Converter4/RConn1
  Simulink-PS Converter2/RConn1 -- Six-Pulse Gate Multiplexer/LConn5
  -/RConn1 -- Converter/RConn2
  Six-Pulse Gate Multiplexer/LConn1 -- Simulink-PS Converter6/RConn1
  +/RConn1 -- Converter/RConn1

== system SimscapeCustomComponents_lib/Microgrid and Renewables/Sources/Wind Plant/Back-to-Back Converters/Switching/Machine Side Converter ==
  mabc : Inport
  Add : Sum
  Constant1 : Constant
  Converter : ee_lib/Semiconductors & Converters/Converters/Converter (Three-Phase)  port_option=ee.enum.threePhasePort.composite  fidelity_option=ee.enum.converters.fidelity.detailed  device_type=ee.enum.converters.switchingdevice.ideal  showThermalPort=false  K=0  Vth=1 V  Vgt=1 V  Vgt_off=-1 V  Ih=1 A  Vf=0.8 V  Ron=0.001 Ohm  Rds=0.001 Ohm  Goff=1e-6 1/Ohm  Eon_scalar=22.86e-3 J  Eoff_scalar=17.14e-3 J  Eoff_natural_commutation=10e-3 J  Voff=300 V  Iout_scalar=600 A  onCurrentMeasDelay=0 s  useCurrentFromPreviousCycle=false  useVoltageFromPreviousCycle=false  diode_param=ee.enum.converters.protectiondiode.nodynamics  diode_Vf=0.01 V  diode_Ron=0.0001 Ohm  diode_Goff=1e-5 1/Ohm  diode_C=50 nF  diode_iRM=-235 A  diode_iF=300 A  diode_idot=-50 A/us  diode_trr_param=ee.enum.converters.diodetrr.trr_factor  diode_trr_factor=3  diode_trr=15 us  diode_Qrr=1500 s*uA  diode_rec_loss_model=ee.enum.diode.reverseRecoveryModel.fixed  diode_ErecVal=0 J  diode_scaleWithIandV=false  diode_ErecMat=zeros(2, 3) J  diode_TjrecVec=[298.15, 398.15] K  diode_IfrecVec=[.1, 1, 10] A  diode_IrecVal=10 A  diode_VrecVal=10 V  diode_tFilter=1 / 1000 / 100 s  thermal_network_parameterization=ee.enum.thermalNetworkTopology.external  Rth=[.08, .5] K/W  Rth_Cauer=[.08, .1, .5] K/W  Rth_Foster=[.08, .14, .22, .16] K/W  thermal_mass_parameterization=ee.enum.thermalNetwork.timeconstant  thermal_mass=[.01, .5] J/K  thermal_mass_Cauer=[.01, .1, .5] J/K  thermal_mass_Foster=[.001, .005, .05, .5] J/K  thermal_time_constant=[.001, .2] s  thermal_time_constant_Cauer=[.001, .1, .2] s  thermal_time_constant_Foster=[7e-05, .0007, .01, .08] s  thermal_mass_initial_temperatures=[25, 25] degC  thermal_mass_initial_temperatures_Cauer=[25, 25, 25] degC  junction_thermal_mass=0.01 J/K  Tvec_initial_Foster=[25, 25, 25, 25] degC  snubber_type=ee.enum.converters.snubber.exclude  Cs=1e-7 F  Rs=0.1 Ohm  Vce_loss=[0, 150, 300] V
  Demux : Demux  Outputs=3
  Demux1 : Demux  Outputs=3
  Gain : Gain  Gain=5
  Gain1 : Gain  Gain=0.5
  PWM Generator : eePwmGenerator/PWM Generator  CarrCount=Up  Tper=1/(fSw*1000)  Tdelay=0  Ts=1/(10*fSw*1000)
  Pulse Generation : Subsystem
  Rate Transition1 : RateTransition  OutPortSampleTime=1/(10*fSw*1000)
  Simulink-PS Converter{1..6} (6 alike) : nesl_utility/Simulink-PS Converter  PhysicalDomain=network_engine_domain  SubClassName=ps_input  LeftPortType=input  RightPortType=output  PseudoPeriodic=off  Frequencies=[]  NoiseDistribution=none  NoiseParameters=[]  Unit=1  AffineConversion=off  FilteringAndDerivatives=provide  SimscapeFilterOrder=1  InputFilterTimeConstant=0.001  UdotUserProvided=0
  Six-Pulse Gate Multiplexer : ee_lib/Semiconductors & Converters/Converters/Six-Pulse Gate Multiplexer  port_option=ee.enum.controlport.ps
  + : PMIOPort  Side=Left
  - : PMIOPort  Port=2  Side=Left
  ~ : PMIOPort  Port=3  Side=Right
  wires:
  [AH] -> Simulink-PS Converter6/1
  mabc/1 -> Add/1
  [CL] -> Simulink-PS Converter1/1
  Demux1/3 -> [CL]
  [CH] -> Simulink-PS Converter2/1
  Demux1/2 -> [BL]
  Add/1 -> Gain1/1
  Demux/1 -> [AH]
  [BL] -> Simulink-PS Converter3/1
  Demux/3 -> [CH]
  [AL] -> Simulink-PS Converter5/1
  Constant1/1 -> Add/2
  PWM Generator/1 -> Gain/1
  Pulse Generation/2(G2) -> Demux1/1
  Pulse Generation/1(G1) -> Demux/1
  Demux/2 -> [BH]
  Gain1/1 -> Rate Transition1/1
  [BH] -> Simulink-PS Converter4/1
  Gain/1 -> Pulse Generation/1(G)
  Rate Transition1/1 -> PWM Generator/1
  Demux1/1 -> [AL]
  connections:
  Six-Pulse Gate Multiplexer/LConn3 -- Simulink-PS Converter4/RConn1
  Simulink-PS Converter1/RConn1 -- Six-Pulse Gate Multiplexer/LConn6
  +/RConn1 -- Converter/RConn1
  Six-Pulse Gate Multiplexer/LConn1 -- Simulink-PS Converter6/RConn1
  -/RConn1 -- Converter/RConn2
  Six-Pulse Gate Multiplexer/LConn4 -- Simulink-PS Converter3/RConn1
  Six-Pulse Gate Multiplexer/LConn2 -- Simulink-PS Converter5/RConn1
  Six-Pulse Gate Multiplexer/RConn1 -- Converter/LConn1
  ~/RConn1 -- Converter/LConn2
  Simulink-PS Converter2/RConn1 -- Six-Pulse Gate Multiplexer/LConn5

== system SimscapeCustomComponents_lib/Microgrid and Renewables/Sources/Wind Plant Integrated/Detailed/PLL/PLL & Measurements1 ==
  V : Inport
  I : Inport  Port=2
  Lead-Lag (Discrete or Continuous) : eeGeneralControl/Lead-Lag (Discrete or Continuous)  T1=0  T2=2e-5  B=inf  A=-inf  init_option=Inherited from block input  x0=0  Ts=Ts
  Subsystem : Subsystem
  Out Bus Element : Outport  PortName=VIbus  Element=Vq
  Out Bus Element1 : Outport  PortName=VIbus  Element=Vd
  Out Bus Element2 : Outport  PortName=VIbus  Element=Freq
  Out Bus Element3 : Outport  PortName=VIbus  Element=Theta
  Out Bus Element4 : Outport  PortName=VIbus  Element=Vmag
  Out Bus Element5 : Outport  PortName=VIbus  Element=Iq
  Out Bus Element6 : Outport  PortName=VIbus  Element=Id
  Out Bus Element7 : Outport  PortName=VIbus  Element=Iabc
  Out Bus Element8 : Outport  PortName=VIbus  Element=Vabc
  wires:
  Subsystem/6(Id1) -> Out Bus Element6/1
  Subsystem/7(Iq1) -> Out Bus Element5/1
  I/1 -> Subsystem/2(Iabc), Lead-Lag (Discrete or Continuous)/1
  Subsystem/1(mag) -> Out Bus Element4/1
  V/1 -> Subsystem/1(Vabc), Out Bus Element8/1
  Subsystem/4(Vd) -> Out Bus Element1/1
  Subsystem/3(angle) -> Out Bus Element3/1
  Subsystem/5(Vq) -> Out Bus Element/1
  Subsystem/2(freq) -> Out Bus Element2/1
  Lead-Lag (Discrete or Continuous)/1 -> Out Bus Element7/1

== system SimscapeCustomComponents_lib/Microgrid and Renewables/Sources/Wind Plant Integrated/Detailed/Wind Turbine and Converters/Signal Conditioning ==
  note: 2
  Bus Element In : Inport  PortName=PMSM  Element=rotorAngle
  BusElementIn2 : Inport  PortName=PMSM  Element=iabc
  BusElementIn3 : Inport  PortName=PMSM  Element=rotorSpeed
  BusElementIn4 : Inport  Port=2  PortName=Meas  Element=windSpeed
  BusElementIn5 : Inport  Port=2  PortName=Meas  Element=Vdc
  Gain : Gain  Gain=-1
  iPMSM : Outport
  rotorSpeed : Outport  Port=2
  theta : Outport  Port=3
  Vdc : Outport  Port=4
  windSpeed : Outport  Port=5
  wires:
  BusElementIn4/1 -> windSpeed/1
  BusElementIn5/1 -> Vdc/1
  Bus Element In/1 -> theta/1
  BusElementIn3/1 -> rotorSpeed/1
  BusElementIn2/1 -> Gain/1
  Gain/1 -> iPMSM/1

== system SimscapeCustomComponents_lib/Microgrid and Renewables/Sources/Wind Plant Integrated/Detailed/Wind Turbine and Converters/Wind Controller ==
  iPMSM : Inport
  w : Inport  Port=2
  theta : Inport  Port=3
  vdc : Inport  Port=4
  Wind speed : Inport  Port=5
  LVRT : Inport  Port=6
  QRef : Inport  Port=7
  VIbus : Inport  Port=8
  Machine Converter Control : Subsystem
  Wind Grid-side Converter Controller : Subsystem
  Chopper Control : Outport
  SM converter control : Outport  Port=2
  m_abc : Outport  Port=3
  wires:
  LVRT/1 -> Wind Grid-side Converter Controller/3(LVRT)
  QRef/1 -> Wind Grid-side Converter Controller/1(QRef)
  VIbus/1 -> Wind Grid-side Converter Controller/2(VIBus)
  w/1 -> Machine Converter Control/2(w_sens)
  Machine Converter Control/2(Chopper Control) -> Chopper Control/1
  theta/1 -> Machine Converter Control/3(a_sens)
  Machine Converter Control/1(SM converter control) -> SM converter control/1
  Wind speed/1 -> Machine Converter Control/5(Wind speed)
  vdc/1 -> Machine Converter Control/4(vdc_sens), Wind Grid-side Converter Controller/4(Vdc)
  iPMSM/1 -> Machine Converter Control/1(iabc_sens)
  Wind Grid-side Converter Controller/2(m_abc) -> m_abc/1
  Wind Grid-side Converter Controller/1(FRT) -> Machine Converter Control/6(LVRT)
